simulink model "LRMate200Experimentor_Dual"  (R2015b)
settings: Solver=FixedStepDiscrete  StartTime=0.0  StopTime=inf  FixedStep=si.SolverTimeStep  RelTol=1e-3  AbsTol=1e-5
undefined symbols (not defined in the file or in its folder): si
libraries: xpcethercatlib x115, slrtlib x16, xpcnilib x10
(part 2 of 2)

== system LRMate200Experimentor_Dual/IO System/DSA System/DSA System 1/EtherCAT DSA TrqLimit ==
  In1 : Inport
  Conversion7 : DataTypeConversion
  Demux : Demux  Outputs=6
  "ToDSA J1TrqLimit " : xpcethercatlib/EtherCAT PDO Transmit   Priority=3  sig_name=Box 1 (Degital Servo Adapter).HS-OUT-AX01.AX01-HSO05  sig_offset=392  sig_type=int16  type_size=16  sig_dim=1  device_id=0  sample_time=0.000250
  ToDSA J2TrqLimit : xpcethercatlib/EtherCAT PDO Transmit   Priority=3  sig_name=Box 1 (Degital Servo Adapter).HS-OUT-AX02.AX02-HSO05  sig_offset=648  sig_type=int16  type_size=16  sig_dim=1  device_id=0  sample_time=0.000250
  ToDSA J3TrqLimit : xpcethercatlib/EtherCAT PDO Transmit   Priority=3  sig_name=Box 1 (Degital Servo Adapter).HS-OUT-AX03.AX03-HSO05  sig_offset=904  sig_type=int16  type_size=16  sig_dim=1  device_id=0  sample_time=0.000250
  ToDSA J4TrqLimit : xpcethercatlib/EtherCAT PDO Transmit   Priority=3  sig_name=Box 1 (Degital Servo Adapter).HS-OUT-AX04.AX04-HSO05  sig_offset=1160  sig_type=int16  type_size=16  sig_dim=1  device_id=0  sample_time=0.000250
  ToDSA J5TrqLimit : xpcethercatlib/EtherCAT PDO Transmit   Priority=3  sig_name=Box 2 (Degital Servo Adapter).HS-OUT-AX01.AX01-HSO05  sig_offset=2696  sig_type=int16  type_size=16  sig_dim=1  device_id=0  sample_time=0.000250
  ToDSA J6TrqLimit : xpcethercatlib/EtherCAT PDO Transmit   Priority=3  sig_name=Box 2 (Degital Servo Adapter).HS-OUT-AX02.AX02-HSO05  sig_offset=2952  sig_type=int16  type_size=16  sig_dim=1  device_id=0  sample_time=0.000250
  wires:
  In1/1 -> Conversion7/1
  Demux/1 -> "ToDSA J1TrqLimit "/1
  Demux/2 -> ToDSA J2TrqLimit/1
  Demux/3 -> ToDSA J3TrqLimit/1
  Demux/4 -> ToDSA J4TrqLimit/1
  Demux/5 -> ToDSA J5TrqLimit/1
  Demux/6 -> ToDSA J6TrqLimit/1
  Conversion7/1 -> Demux/1

== system LRMate200Experimentor_Dual/IO System/DSA System/DSA System 1/EtherCAT DSA VelOut ==
  FromDSA J1Vel : xpcethercatlib/EtherCAT PDO Receive  Priority=2  sig_name=Box 1 (Degital Servo Adapter).HS-IN-AX01.AX01-HSI10  sig_offset=472  sig_type=int32  type_size=32  sig_dim=1  device_id=0  sample_time=0.000250
  FromDSA J2Vel : xpcethercatlib/EtherCAT PDO Receive  Priority=2  sig_name=Box 1 (Degital Servo Adapter).HS-IN-AX02.AX02-HSI10  sig_offset=728  sig_type=int32  type_size=32  sig_dim=1  device_id=0  sample_time=0.000250
  FromDSA J3Vel : xpcethercatlib/EtherCAT PDO Receive  Priority=2  sig_name=Box 1 (Degital Servo Adapter).HS-IN-AX03.AX03-HSI10  sig_offset=984  sig_type=int32  type_size=32  sig_dim=1  device_id=0  sample_time=0.000250
  FromDSA J4Vel : xpcethercatlib/EtherCAT PDO Receive  Priority=2  sig_name=Box 1 (Degital Servo Adapter).HS-IN-AX04.AX04-HSI10  sig_offset=1240  sig_type=int32  type_size=32  sig_dim=1  device_id=0  sample_time=0.000250
  FromDSA J5Vel : xpcethercatlib/EtherCAT PDO Receive  Priority=2  sig_name=Box 2 (Degital Servo Adapter).HS-IN-AX01.AX01-HSI10  sig_offset=2776  sig_type=int32  type_size=32  sig_dim=1  device_id=0  sample_time=0.000250
  FromDSA J6Vel : xpcethercatlib/EtherCAT PDO Receive  Priority=2  sig_name=Box 2 (Degital Servo Adapter).HS-IN-AX02.AX02-HSI10  sig_offset=3032  sig_type=int32  type_size=32  sig_dim=1  device_id=0  sample_time=0.000250
  Mux : Mux  Inputs=6
  Rate Transition : RateTransition  OutPortSampleTime=si.tsv
  VelOut : Outport
  wires:
  FromDSA J6Vel/1 -> Mux/6
  FromDSA J4Vel/1 -> Mux/4
  FromDSA J2Vel/1 -> Mux/2
  FromDSA J5Vel/1 -> Mux/5
  FromDSA J3Vel/1 -> Mux/3
  FromDSA J1Vel/1 -> Mux/1
  Rate Transition/1 -> VelOut/1
  Mux/1 -> Rate Transition/1

== system LRMate200Experimentor_Dual/IO System/DSA System/DSA System 2/EtherCAT DSA AxEtcInfo ==
  FromDSA J1AxEtcInfo : xpcethercatlib/EtherCAT PDO Receive  Priority=2  sig_name=Box 3 (Degital Servo Adapter).NS-IN-AX01.AX01-NSI07  sig_offset=6312  sig_type=uint16  type_size=16  sig_dim=1  device_id=0  sample_time=0.000250
  FromDSA J2AxEtcInfo : xpcethercatlib/EtherCAT PDO Receive  Priority=2  sig_name=Box 3 (Degital Servo Adapter).NS-IN-AX02.AX02-NSI07  sig_offset=6504  sig_type=uint16  type_size=16  sig_dim=1  device_id=0  sample_time=0.000250
  FromDSA J3AxEtcInfo : xpcethercatlib/EtherCAT PDO Receive  Priority=2  sig_name=Box 3 (Degital Servo Adapter).NS-IN-AX03.AX03-NSI07  sig_offset=6696  sig_type=uint16  type_size=16  sig_dim=1  device_id=0  sample_time=0.000250
  FromDSA J4AxEtcInfo : xpcethercatlib/EtherCAT PDO Receive  Priority=2  sig_name=Box 3 (Degital Servo Adapter).NS-IN-AX04.AX04-NSI07  sig_offset=6888  sig_type=uint16  type_size=16  sig_dim=1  device_id=0  sample_time=0.000250
  FromDSA J5AxEtcInfo : xpcethercatlib/EtherCAT PDO Receive  Priority=2  sig_name=Box 4 (Degital Servo Adapter).NS-IN-AX01.AX01-NSI07  sig_offset=8616  sig_type=uint16  type_size=16  sig_dim=1  device_id=0  sample_time=0.000250
  FromDSA J6AxEtcInfo : xpcethercatlib/EtherCAT PDO Receive  Priority=2  sig_name=Box 4 (Degital Servo Adapter).NS-IN-AX02.AX02-NSI07  sig_offset=8808  sig_type=uint16  type_size=16  sig_dim=1  device_id=0  sample_time=0.000250
  Mux : Mux  Inputs=6
  Rate Transition : RateTransition  OutPortSampleTime=si.tsv
  AxEtcInfoOut : Outport
  wires:
  FromDSA J6AxEtcInfo/1 -> Mux/6
  FromDSA J4AxEtcInfo/1 -> Mux/4
  FromDSA J2AxEtcInfo/1 -> Mux/2
  FromDSA J5AxEtcInfo/1 -> Mux/5
  FromDSA J3AxEtcInfo/1 -> Mux/3
  FromDSA J1AxEtcInfo/1 -> Mux/1
  Mux/1 -> Rate Transition/1
  Rate Transition/1 -> AxEtcInfoOut/1

== system LRMate200Experimentor_Dual/IO System/DSA System/DSA System 2/EtherCAT DSA CurrentOut ==
  FromDSA J1Current : xpcethercatlib/EtherCAT PDO Receive  Priority=2  sig_name=Box 3 (Degital Servo Adapter).HS-IN-AX01.AX01-HSI03  sig_offset=4968  sig_type=int16  type_size=16  sig_dim=1  device_id=0  sample_time=0.000250
  FromDSA J2Current : xpcethercatlib/EtherCAT PDO Receive  Priority=2  sig_name=Box 3 (Degital Servo Adapter).HS-IN-AX02.AX02-HSI03  sig_offset=5224  sig_type=int16  type_size=16  sig_dim=1  device_id=0  sample_time=0.000250
  FromDSA J3Current : xpcethercatlib/EtherCAT PDO Receive  Priority=2  sig_name=Box 3 (Degital Servo Adapter).HS-IN-AX03.AX03-HSI03  sig_offset=5480  sig_type=int16  type_size=16  sig_dim=1  device_id=0  sample_time=0.000250
  FromDSA J4Current : xpcethercatlib/EtherCAT PDO Receive  Priority=2  sig_name=Box 3 (Degital Servo Adapter).HS-IN-AX04.AX04-HSI03  sig_offset=5736  sig_type=int16  type_size=16  sig_dim=1  device_id=0  sample_time=0.000250
  FromDSA J5Current : xpcethercatlib/EtherCAT PDO Receive  Priority=2  sig_name=Box 4 (Degital Servo Adapter).HS-IN-AX01.AX01-HSI03  sig_offset=7272  sig_type=int16  type_size=16  sig_dim=1  device_id=0  sample_time=0.000250
  FromDSA J6Current : xpcethercatlib/EtherCAT PDO Receive  Priority=2  sig_name=Box 4 (Degital Servo Adapter).HS-IN-AX02.AX02-HSI03  sig_offset=7528  sig_type=int16  type_size=16  sig_dim=1  device_id=0  sample_time=0.000250
  Mux : Mux  Inputs=6
  Rate Transition : RateTransition  OutPortSampleTime=si.tsv
  CurrentOut : Outport
  wires:
  FromDSA J6Current/1 -> Mux/6
  FromDSA J4Current/1 -> Mux/4
  FromDSA J2Current/1 -> Mux/2
  FromDSA J5Current/1 -> Mux/5
  FromDSA J3Current/1 -> Mux/3
  FromDSA J1Current/1 -> Mux/1
  Mux/1 -> Rate Transition/1
  Rate Transition/1 -> CurrentOut/1

== system LRMate200Experimentor_Dual/IO System/DSA System/DSA System 2/EtherCAT DSA IniPos ==
  FromDSA J1IniPos : xpcethercatlib/EtherCAT PDO Receive  Priority=2  sig_name=Box 3 (Degital Servo Adapter).NS-IN-AX01.AX01-NSI02  sig_offset=6232  sig_type=int32  type_size=32  sig_dim=1  device_id=0  sample_time=0.000250
  FromDSA J2IniPos : xpcethercatlib/EtherCAT PDO Receive  Priority=2  sig_name=Box 3 (Degital Servo Adapter).NS-IN-AX02.AX02-NSI02  sig_offset=6424  sig_type=int32  type_size=32  sig_dim=1  device_id=0  sample_time=0.000250
  FromDSA J3IniPos : xpcethercatlib/EtherCAT PDO Receive  Priority=2  sig_name=Box 3 (Degital Servo Adapter).NS-IN-AX03.AX03-NSI02  sig_offset=6616  sig_type=int32  type_size=32  sig_dim=1  device_id=0  sample_time=0.000250
  FromDSA J4IniPos : xpcethercatlib/EtherCAT PDO Receive  Priority=2  sig_name=Box 3 (Degital Servo Adapter).NS-IN-AX04.AX04-NSI02  sig_offset=6808  sig_type=int32  type_size=32  sig_dim=1  device_id=0  sample_time=0.000250
  FromDSA J5IniPos : xpcethercatlib/EtherCAT PDO Receive  Priority=2  sig_name=Box 4 (Degital Servo Adapter).NS-IN-AX01.AX01-NSI02  sig_offset=8536  sig_type=int32  type_size=32  sig_dim=1  device_id=0  sample_time=0.000250
  FromDSA J6IniPos : xpcethercatlib/EtherCAT PDO Receive  Priority=2  sig_name=Box 4 (Degital Servo Adapter).NS-IN-AX02.AX02-NSI02  sig_offset=8728  sig_type=int32  type_size=32  sig_dim=1  device_id=0  sample_time=0.000250
  Mux : Mux  Inputs=6
  Rate Transition : RateTransition  OutPortSampleTime=si.tsv
  ini_pos : Outport
  wires:
  FromDSA J6IniPos/1 -> Mux/6
  FromDSA J4IniPos/1 -> Mux/4
  FromDSA J2IniPos/1 -> Mux/2
  FromDSA J5IniPos/1 -> Mux/5
  FromDSA J3IniPos/1 -> Mux/3
  FromDSA J1IniPos/1 -> Mux/1
  Mux/1 -> Rate Transition/1
  Rate Transition/1 -> ini_pos/1

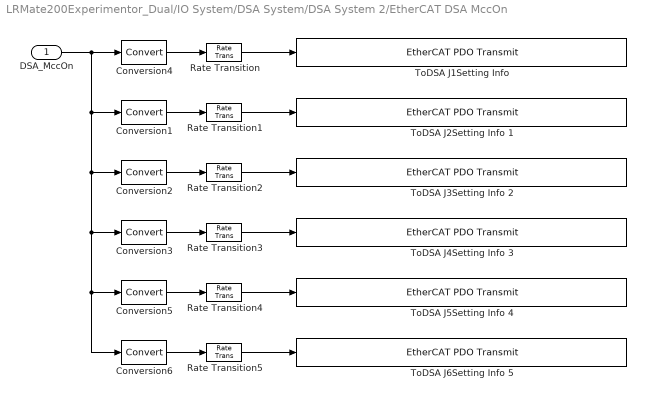
== system LRMate200Experimentor_Dual/IO System/DSA System/DSA System 2/EtherCAT DSA MccOn ==
  DSA_MccOn : Inport
  Conversion{1..6} (6 alike) : DataTypeConversion
  Rate Transition{,1..5} (6 alike) : RateTransition
  "ToDSA J1Setting Info " : xpcethercatlib/EtherCAT PDO Transmit   Priority=3  sig_name=Box 3 (Degital Servo Adapter).NS-OUT-AX01.AX01-NSO03  sig_offset=6248  sig_type=uint16  type_size=16  sig_dim=1  device_id=0  sample_time=0.000250
  ToDSA J2Setting Info 1 : xpcethercatlib/EtherCAT PDO Transmit   Priority=3  sig_name=Box 3 (Degital Servo Adapter).NS-OUT-AX02.AX02-NSO03  sig_offset=6504  sig_type=uint16  type_size=16  sig_dim=1  device_id=0  sample_time=0.000250
  ToDSA J3Setting Info 2 : xpcethercatlib/EtherCAT PDO Transmit   Priority=3  sig_name=Box 3 (Degital Servo Adapter).NS-OUT-AX03.AX03-NSO03  sig_offset=6760  sig_type=uint16  type_size=16  sig_dim=1  device_id=0  sample_time=0.000250
  ToDSA J4Setting Info 3 : xpcethercatlib/EtherCAT PDO Transmit   Priority=3  sig_name=Box 3 (Degital Servo Adapter).NS-OUT-AX04.AX04-NSO03  sig_offset=7016  sig_type=uint16  type_size=16  sig_dim=1  device_id=0  sample_time=0.000250
  ToDSA J5Setting Info 4 : xpcethercatlib/EtherCAT PDO Transmit   Priority=3  sig_name=Box 4 (Degital Servo Adapter).NS-OUT-AX01.AX01-NSO03  sig_offset=8552  sig_type=uint16  type_size=16  sig_dim=1  device_id=0  sample_time=0.000250
  ToDSA J6Setting Info 5 : xpcethercatlib/EtherCAT PDO Transmit   Priority=3  sig_name=Box 4 (Degital Servo Adapter).NS-OUT-AX02.AX02-NSO03  sig_offset=8808  sig_type=uint16  type_size=16  sig_dim=1  device_id=0  sample_time=0.000250
  wires:
  Rate Transition/1 -> "ToDSA J1Setting Info "/1
  Conversion4/1 -> Rate Transition/1
  DSA_MccOn/1 -> Conversion6/1, Conversion5/1, Conversion3/1, Conversion2/1, Conversion1/1, Conversion4/1
  Rate Transition1/1 -> ToDSA J2Setting Info 1/1
  Conversion1/1 -> Rate Transition1/1
  Rate Transition2/1 -> ToDSA J3Setting Info 2/1
  Conversion2/1 -> Rate Transition2/1
  Rate Transition3/1 -> ToDSA J4Setting Info 3/1
  Conversion3/1 -> Rate Transition3/1
  Rate Transition4/1 -> ToDSA J5Setting Info 4/1
  Conversion5/1 -> Rate Transition4/1
  Rate Transition5/1 -> ToDSA J6Setting Info 5/1
  Conversion6/1 -> Rate Transition5/1

== system LRMate200Experimentor_Dual/IO System/DSA System/DSA System 2/EtherCAT DSA PosOut ==
  FromDSA J1Pos : xpcethercatlib/EtherCAT PDO Receive  Priority=2  sig_name=Box 3 (Degital Servo Adapter).HS-IN-AX01.AX01-HSI12  sig_offset=5112  sig_type=int32  type_size=32  sig_dim=1  device_id=0  sample_time=0.000250
  FromDSA J2Pos : xpcethercatlib/EtherCAT PDO Receive  Priority=2  sig_name=Box 3 (Degital Servo Adapter).HS-IN-AX02.AX02-HSI12  sig_offset=5368  sig_type=int32  type_size=32  sig_dim=1  device_id=0  sample_time=0.000250
  FromDSA J3Pos : xpcethercatlib/EtherCAT PDO Receive  Priority=2  sig_name=Box 3 (Degital Servo Adapter).HS-IN-AX03.AX03-HSI12  sig_offset=5624  sig_type=int32  type_size=32  sig_dim=1  device_id=0  sample_time=0.000250
  FromDSA J4Pos : xpcethercatlib/EtherCAT PDO Receive  Priority=2  sig_name=Box 3 (Degital Servo Adapter).HS-IN-AX04.AX04-HSI12  sig_offset=5880  sig_type=int32  type_size=32  sig_dim=1  device_id=0  sample_time=0.000250
  FromDSA J5Pos : xpcethercatlib/EtherCAT PDO Receive  Priority=2  sig_name=Box 4 (Degital Servo Adapter).HS-IN-AX01.AX01-HSI12  sig_offset=7416  sig_type=int32  type_size=32  sig_dim=1  device_id=0  sample_time=0.000250
  FromDSA J6Pos : xpcethercatlib/EtherCAT PDO Receive  Priority=2  sig_name=Box 4 (Degital Servo Adapter).HS-IN-AX02.AX02-HSI12  sig_offset=7672  sig_type=int32  type_size=32  sig_dim=1  device_id=0  sample_time=0.000250
  Mux : Mux  Inputs=6
  Rate Transition : RateTransition  OutPortSampleTime=si.tsv
  PosOut : Outport
  wires:
  FromDSA J6Pos/1 -> Mux/6
  FromDSA J4Pos/1 -> Mux/4
  FromDSA J2Pos/1 -> Mux/2
  FromDSA J5Pos/1 -> Mux/5
  FromDSA J3Pos/1 -> Mux/3
  FromDSA J1Pos/1 -> Mux/1
  Mux/1 -> Rate Transition/1
  Rate Transition/1 -> PosOut/1

== system LRMate200Experimentor_Dual/IO System/DSA System/DSA System 2/EtherCAT DSA TrqCmd ==
  In1 : Inport
  Conversion1 : DataTypeConversion
  Demux : Demux  Outputs=6
  Rate Transition : RateTransition
  "ToDSA J1TrqCmd " : xpcethercatlib/EtherCAT PDO Transmit   Priority=3  sig_name=Box 3 (Degital Servo Adapter).HS-OUT-AX01.AX01-HSO04  sig_offset=4984  sig_type=int16  type_size=16  sig_dim=1  device_id=0  sample_time=0.000250
  ToDSA J2TrqCmd : xpcethercatlib/EtherCAT PDO Transmit   Priority=3  sig_name=Box 3 (Degital Servo Adapter).HS-OUT-AX02.AX02-HSO04  sig_offset=5240  sig_type=int16  type_size=16  sig_dim=1  device_id=0  sample_time=0.000250
  ToDSA J3TrqCmd : xpcethercatlib/EtherCAT PDO Transmit   Priority=3  sig_name=Box 3 (Degital Servo Adapter).HS-OUT-AX03.AX03-HSO04  sig_offset=5496  sig_type=int16  type_size=16  sig_dim=1  device_id=0  sample_time=0.000250
  ToDSA J4TrqCmd : xpcethercatlib/EtherCAT PDO Transmit   Priority=3  sig_name=Box 3 (Degital Servo Adapter).HS-OUT-AX04.AX04-HSO04  sig_offset=5752  sig_type=int16  type_size=16  sig_dim=1  device_id=0  sample_time=0.000250
  ToDSA J5TrqCmd : xpcethercatlib/EtherCAT PDO Transmit   Priority=3  sig_name=Box 4 (Degital Servo Adapter).HS-OUT-AX01.AX01-HSO04  sig_offset=7288  sig_type=int16  type_size=16  sig_dim=1  device_id=0  sample_time=0.000250
  ToDSA J6TrqCmd : xpcethercatlib/EtherCAT PDO Transmit   Priority=3  sig_name=Box 4 (Degital Servo Adapter).HS-OUT-AX02.AX02-HSO04  sig_offset=7544  sig_type=int16  type_size=16  sig_dim=1  device_id=0  sample_time=0.000250
  wires:
  In1/1 -> Conversion1/1
  Conversion1/1 -> Rate Transition/1
  Rate Transition/1 -> Demux/1
  Demux/1 -> "ToDSA J1TrqCmd "/1
  Demux/2 -> ToDSA J2TrqCmd/1
  Demux/3 -> ToDSA J3TrqCmd/1
  Demux/4 -> ToDSA J4TrqCmd/1
  Demux/5 -> ToDSA J5TrqCmd/1
  Demux/6 -> ToDSA J6TrqCmd/1

== system LRMate200Experimentor_Dual/IO System/DSA System/DSA System 2/EtherCAT DSA TrqCmdOut ==
  FromDSA J1TrqCmd : xpcethercatlib/EtherCAT PDO Receive  Priority=2  sig_name=Box 3 (Degital Servo Adapter).HS-IN-AX01.AX01-HSI02  sig_offset=4952  sig_type=int16  type_size=16  sig_dim=1  device_id=0  sample_time=0.000250
  FromDSA J2TrqCmd : xpcethercatlib/EtherCAT PDO Receive  Priority=2  sig_name=Box 3 (Degital Servo Adapter).HS-IN-AX02.AX02-HSI02  sig_offset=5208  sig_type=int16  type_size=16  sig_dim=1  device_id=0  sample_time=0.000250
  FromDSA J3TrqCmd2 : xpcethercatlib/EtherCAT PDO Receive  Priority=2  sig_name=Box 3 (Degital Servo Adapter).HS-IN-AX03.AX03-HSI02  sig_offset=5464  sig_type=int16  type_size=16  sig_dim=1  device_id=0  sample_time=0.000250
  FromDSA J4TrqCmd3 : xpcethercatlib/EtherCAT PDO Receive  Priority=2  sig_name=Box 3 (Degital Servo Adapter).HS-IN-AX04.AX04-HSI02  sig_offset=5720  sig_type=int16  type_size=16  sig_dim=1  device_id=0  sample_time=0.000250
  FromDSA J5TrqCmd4 : xpcethercatlib/EtherCAT PDO Receive  Priority=2  sig_name=Box 4 (Degital Servo Adapter).HS-IN-AX01.AX01-HSI02  sig_offset=7256  sig_type=int16  type_size=16  sig_dim=1  device_id=0  sample_time=0.000250
  FromDSA J6TrqCmd5 : xpcethercatlib/EtherCAT PDO Receive  Priority=2  sig_name=Box 4 (Degital Servo Adapter).HS-IN-AX02.AX02-HSI02  sig_offset=7512  sig_type=int16  type_size=16  sig_dim=1  device_id=0  sample_time=0.000250
  Mux : Mux  Inputs=6
  Rate Transition : RateTransition  OutPortSampleTime=si.tsv
  TrqCmdOut : Outport
  wires:
  FromDSA J6TrqCmd5/1 -> Mux/6
  FromDSA J4TrqCmd3/1 -> Mux/4
  FromDSA J2TrqCmd/1 -> Mux/2
  FromDSA J5TrqCmd4/1 -> Mux/5
  FromDSA J3TrqCmd2/1 -> Mux/3
  FromDSA J1TrqCmd/1 -> Mux/1
  Mux/1 -> Rate Transition/1
  Rate Transition/1 -> TrqCmdOut/1

== system LRMate200Experimentor_Dual/IO System/DSA System/DSA System 2/EtherCAT DSA TrqLimit ==
  In1 : Inport
  Conversion1 : DataTypeConversion
  Demux : Demux  Outputs=6
  "ToDSA J1TrqLimit " : xpcethercatlib/EtherCAT PDO Transmit   Priority=3  sig_name=Box 3 (Degital Servo Adapter).HS-OUT-AX01.AX01-HSO05  sig_offset=5000  sig_type=int16  type_size=16  sig_dim=1  device_id=0  sample_time=0.000250
  ToDSA J2TrqLimit : xpcethercatlib/EtherCAT PDO Transmit   Priority=3  sig_name=Box 3 (Degital Servo Adapter).HS-OUT-AX02.AX02-HSO05  sig_offset=5256  sig_type=int16  type_size=16  sig_dim=1  device_id=0  sample_time=0.000250
  ToDSA J3TrqLimit : xpcethercatlib/EtherCAT PDO Transmit   Priority=3  sig_name=Box 3 (Degital Servo Adapter).HS-OUT-AX03.AX03-HSO05  sig_offset=5512  sig_type=int16  type_size=16  sig_dim=1  device_id=0  sample_time=0.000250
  ToDSA J4TrqLimit : xpcethercatlib/EtherCAT PDO Transmit   Priority=3  sig_name=Box 3 (Degital Servo Adapter).HS-OUT-AX04.AX04-HSO05  sig_offset=5768  sig_type=int16  type_size=16  sig_dim=1  device_id=0  sample_time=0.000250
  ToDSA J5TrqLimit : xpcethercatlib/EtherCAT PDO Transmit   Priority=3  sig_name=Box 4 (Degital Servo Adapter).HS-OUT-AX01.AX01-HSO05  sig_offset=7304  sig_type=int16  type_size=16  sig_dim=1  device_id=0  sample_time=0.000250
  ToDSA J6TrqLimit : xpcethercatlib/EtherCAT PDO Transmit   Priority=3  sig_name=Box 4 (Degital Servo Adapter).HS-OUT-AX02.AX02-HSO05  sig_offset=7560  sig_type=int16  type_size=16  sig_dim=1  device_id=0  sample_time=0.000250
  wires:
  In1/1 -> Conversion1/1
  Conversion1/1 -> Demux/1
  Demux/1 -> "ToDSA J1TrqLimit "/1
  Demux/2 -> ToDSA J2TrqLimit/1
  Demux/3 -> ToDSA J3TrqLimit/1
  Demux/4 -> ToDSA J4TrqLimit/1
  Demux/5 -> ToDSA J5TrqLimit/1
  Demux/6 -> ToDSA J6TrqLimit/1

== system LRMate200Experimentor_Dual/IO System/DSA System/DSA System 2/EtherCAT DSA VelOut ==
  FromDSA J1Vel : xpcethercatlib/EtherCAT PDO Receive  Priority=2  sig_name=Box 3 (Degital Servo Adapter).HS-IN-AX01.AX01-HSI10  sig_offset=5080  sig_type=int32  type_size=32  sig_dim=1  device_id=0  sample_time=0.000250
  FromDSA J2Vel : xpcethercatlib/EtherCAT PDO Receive  Priority=2  sig_name=Box 3 (Degital Servo Adapter).HS-IN-AX02.AX02-HSI10  sig_offset=5336  sig_type=int32  type_size=32  sig_dim=1  device_id=0  sample_time=0.000250
  FromDSA J3Vel : xpcethercatlib/EtherCAT PDO Receive  Priority=2  sig_name=Box 3 (Degital Servo Adapter).HS-IN-AX03.AX03-HSI10  sig_offset=5592  sig_type=int32  type_size=32  sig_dim=1  device_id=0  sample_time=0.000250
  FromDSA J4Vel : xpcethercatlib/EtherCAT PDO Receive  Priority=2  sig_name=Box 3 (Degital Servo Adapter).HS-IN-AX04.AX04-HSI10  sig_offset=5848  sig_type=int32  type_size=32  sig_dim=1  device_id=0  sample_time=0.000250
  FromDSA J5Vel : xpcethercatlib/EtherCAT PDO Receive  Priority=2  sig_name=Box 4 (Degital Servo Adapter).HS-IN-AX01.AX01-HSI10  sig_offset=7384  sig_type=int32  type_size=32  sig_dim=1  device_id=0  sample_time=0.000250
  FromDSA J6Vel : xpcethercatlib/EtherCAT PDO Receive  Priority=2  sig_name=Box 4 (Degital Servo Adapter).HS-IN-AX02.AX02-HSI10  sig_offset=7640  sig_type=int32  type_size=32  sig_dim=1  device_id=0  sample_time=0.000250
  Mux : Mux  Inputs=6
  Rate Transition : RateTransition  OutPortSampleTime=si.tsv
  VelOut : Outport
  wires:
  FromDSA J6Vel/1 -> Mux/6
  FromDSA J4Vel/1 -> Mux/4
  FromDSA J2Vel/1 -> Mux/2
  FromDSA J5Vel/1 -> Mux/5
  FromDSA J3Vel/1 -> Mux/3
  FromDSA J1Vel/1 -> Mux/1
  Rate Transition/1 -> VelOut/1
  Mux/1 -> Rate Transition/1

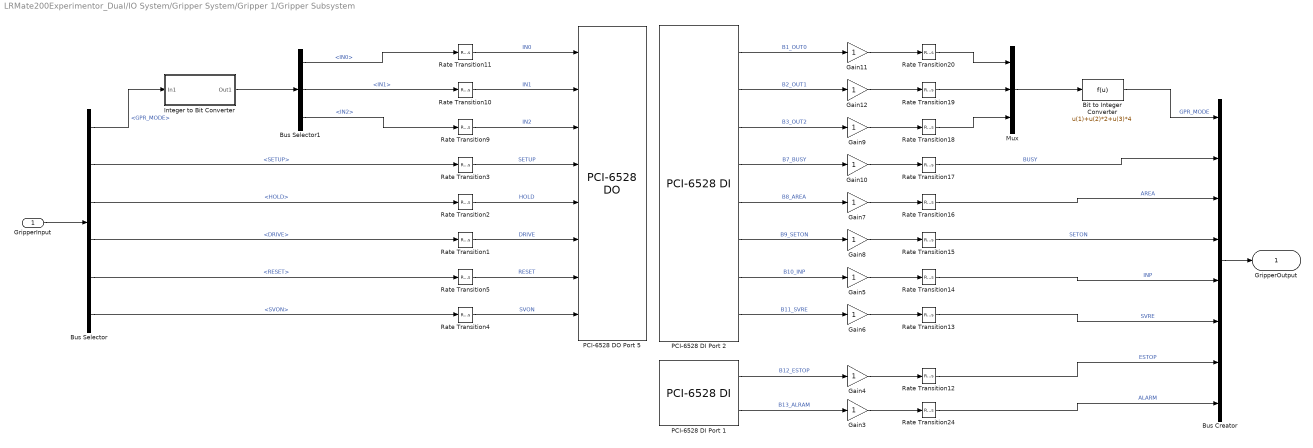
== system LRMate200Experimentor_Dual/IO System/Gripper System/Gripper 1/Gripper Subsystem ==
  GripperInput : Inport
  Bit to Integer Converter : Fcn  Expr=u(1)+u(2)*2+u(3)*4
  Bus Creator : BusCreator  Inputs=8
  Bus Selector : BusSelector  OutputSignals=GPR_MODE,SETUP,HOLD,DRIVE,RESET,SVON
  Bus Selector1 : BusSelector  OutputSignals=IN0,IN1,IN2
  Gain{3..12} (10 alike) : Gain
  Integer to Bit Converter : Subsystem  TreatAsAtomicUnit=on
  Mux : Mux  Inputs=3
  PCI-6528 DI Port 1 : xpcnilib/Digital Input/PCI-6528 DI  channel=[8 7]  port=B  filter=[0]  filtertime=0  sample=.001  slot=-1
  PCI-6528 DI Port 2 : xpcnilib/Digital Input/PCI-6528 DI  channel=[8 7 6 5 4 3 2 1]  port=C  filter=[0]  filtertime=0  sample=.001  slot=-1
  PCI-6528 DO Port 5 : xpcnilib/Digital Output/PCI-6528 DO  channel=[8 7 6 5 4 3 2 1]  port=C  reset=[1]  initValue=[0]  sample=0.001  slot=-1
  Rate Transition{1..5,9..20,24} (18 alike) : RateTransition  OutPortSampleTime=si.tsv
  GripperOutput : Outport
  wires:
  Bus Selector/4 -> Rate Transition1/1  "<DRIVE>"
  Rate Transition4/1 -> PCI-6528 DO Port 5/8  "SVON"
  Rate Transition1/1 -> PCI-6528 DO Port 5/6  "DRIVE"
  Rate Transition3/1 -> PCI-6528 DO Port 5/4  "SETUP"
  Bus Selector1/1 -> Rate Transition11/1  "<IN0>"
  Bus Selector1/2 -> Rate Transition10/1  "<IN1>"
  Bus Selector1/3 -> Rate Transition9/1  "<IN2>"
  Bus Selector/2 -> Rate Transition3/1  "<SETUP>"
  Bus Selector/3 -> Rate Transition2/1  "<HOLD>"
  Bus Selector/6 -> Rate Transition4/1  "<SVON>"
  Bus Selector/5 -> Rate Transition5/1  "<RESET>"
  Rate Transition2/1 -> PCI-6528 DO Port 5/5  "HOLD"
  Rate Transition9/1 -> PCI-6528 DO Port 5/3  "IN2"
  Rate Transition10/1 -> PCI-6528 DO Port 5/2  "IN1"
  Rate Transition11/1 -> PCI-6528 DO Port 5/1  "IN0"
  Rate Transition5/1 -> PCI-6528 DO Port 5/7  "RESET"
  GripperInput/1 -> Bus Selector/1
  Gain3/1 -> Rate Transition24/1
  PCI-6528 DI Port 2/6 -> Gain8/1  "B9_SETON"
  Bus Creator/1 -> GripperOutput/1
  Mux/1 -> Bit to Integer Converter/1
  Rate Transition18/1 -> Mux/3
  PCI-6528 DI Port 1/1 -> Gain4/1  "B12_ESTOP"
  PCI-6528 DI Port 2/3 -> Gain9/1  "B3_OUT2"
  PCI-6528 DI Port 2/4 -> Gain10/1  "B7_BUSY"
  Rate Transition20/1 -> Mux/1
  Rate Transition19/1 -> Mux/2
  PCI-6528 DI Port 2/2 -> Gain12/1  "B2_OUT1"
  Gain8/1 -> Rate Transition15/1
  Gain7/1 -> Rate Transition16/1
  PCI-6528 DI Port 2/5 -> Gain7/1  "B8_AREA"
  PCI-6528 DI Port 1/2 -> Gain3/1  "B13_ALRAM"
  Gain11/1 -> Rate Transition20/1
  Gain9/1 -> Rate Transition18/1
  Gain10/1 -> Rate Transition17/1
  Gain12/1 -> Rate Transition19/1
  Gain4/1 -> Rate Transition12/1
  Gain6/1 -> Rate Transition13/1
  PCI-6528 DI Port 2/8 -> Gain6/1  "B11_SVRE"
  PCI-6528 DI Port 2/7 -> Gain5/1  "B10_INP"
  Gain5/1 -> Rate Transition14/1
  PCI-6528 DI Port 2/1 -> Gain11/1  "B1_OUT0"
  Rate Transition16/1 -> Bus Creator/3  "AREA"
  Rate Transition17/1 -> Bus Creator/2  "BUSY"
  Rate Transition15/1 -> Bus Creator/4  "SETON"
  Bit to Integer Converter/1 -> Bus Creator/1  "GPR_MODE"
  Rate Transition13/1 -> Bus Creator/6  "SVRE"
  Rate Transition14/1 -> Bus Creator/5  "INP"
  Rate Transition12/1 -> Bus Creator/7  "ESTOP"
  Rate Transition24/1 -> Bus Creator/8  "ALARM"
  Bus Selector/1 -> Integer to Bit Converter/1(In1)  "<GPR_MODE>"
  Integer to Bit Converter/1(Out1) -> Bus Selector1/1

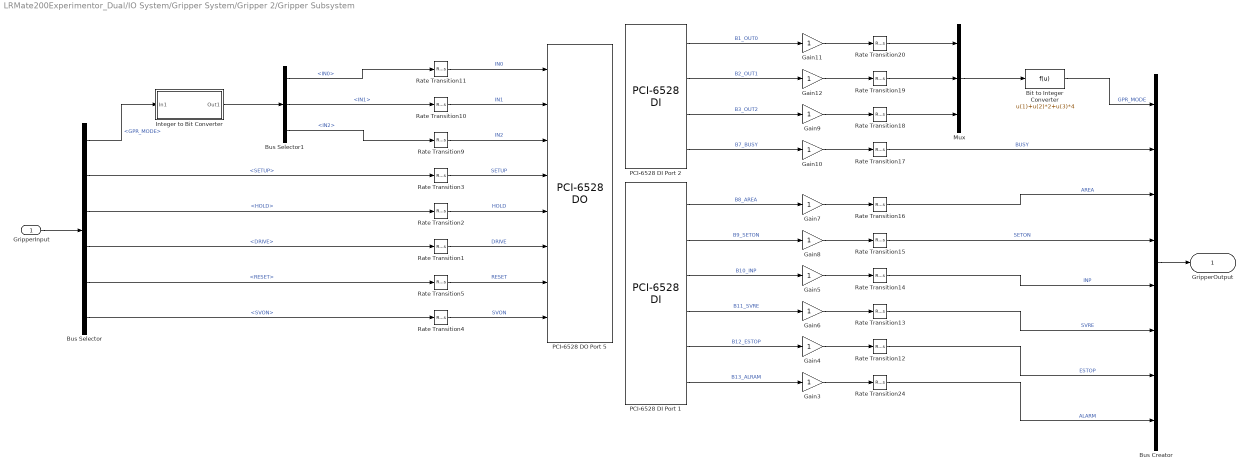
== system LRMate200Experimentor_Dual/IO System/Gripper System/Gripper 2/Gripper Subsystem ==
  GripperInput : Inport
  Bit to Integer Converter : Fcn  Expr=u(1)+u(2)*2+u(3)*4
  Bus Creator : BusCreator  Inputs=8
  Bus Selector : BusSelector  OutputSignals=GPR_MODE,SETUP,HOLD,DRIVE,RESET,SVON
  Bus Selector1 : BusSelector  OutputSignals=IN0,IN1,IN2
  Gain{3..12} (10 alike) : Gain
  Integer to Bit Converter : Subsystem  TreatAsAtomicUnit=on
  Mux : Mux  Inputs=3
  PCI-6528 DI Port 1 : xpcnilib/Digital Input/PCI-6528 DI  channel=[8 7 6 5 4 3]  port=A  filter=[0]  filtertime=0  sample=.001  slot=-1
  PCI-6528 DI Port 2 : xpcnilib/Digital Input/PCI-6528 DI  channel=[4 3 2 1]  port=B  filter=[0]  filtertime=0  sample=.001  slot=-1
  PCI-6528 DO Port 5 : xpcnilib/Digital Output/PCI-6528 DO  channel=[8 7 6 5 4 3 2 1]  port=B  reset=[1]  initValue=[0]  sample=0.001  slot=-1
  Rate Transition{1..5,9..20,24} (18 alike) : RateTransition  OutPortSampleTime=si.tsv
  GripperOutput : Outport
  wires:
  Bus Selector/4 -> Rate Transition1/1  "<DRIVE>"
  Rate Transition4/1 -> PCI-6528 DO Port 5/8  "SVON"
  Rate Transition1/1 -> PCI-6528 DO Port 5/6  "DRIVE"
  Rate Transition3/1 -> PCI-6528 DO Port 5/4  "SETUP"
  Bus Selector/2 -> Rate Transition3/1  "<SETUP>"
  Bus Selector/3 -> Rate Transition2/1  "<HOLD>"
  Bus Selector/6 -> Rate Transition4/1  "<SVON>"
  Bus Selector/5 -> Rate Transition5/1  "<RESET>"
  Rate Transition2/1 -> PCI-6528 DO Port 5/5  "HOLD"
  Rate Transition9/1 -> PCI-6528 DO Port 5/3  "IN2"
  Rate Transition10/1 -> PCI-6528 DO Port 5/2  "IN1"
  Rate Transition11/1 -> PCI-6528 DO Port 5/1  "IN0"
  Rate Transition5/1 -> PCI-6528 DO Port 5/7  "RESET"
  GripperInput/1 -> Bus Selector/1
  Gain3/1 -> Rate Transition24/1
  PCI-6528 DI Port 1/2 -> Gain8/1  "B9_SETON"
  Bus Creator/1 -> GripperOutput/1
  Mux/1 -> Bit to Integer Converter/1
  Rate Transition18/1 -> Mux/3
  PCI-6528 DI Port 1/5 -> Gain4/1  "B12_ESTOP"
  PCI-6528 DI Port 2/3 -> Gain9/1  "B3_OUT2"
  PCI-6528 DI Port 2/4 -> Gain10/1  "B7_BUSY"
  Rate Transition20/1 -> Mux/1
  Rate Transition19/1 -> Mux/2
  PCI-6528 DI Port 2/2 -> Gain12/1  "B2_OUT1"
  Gain8/1 -> Rate Transition15/1
  Gain7/1 -> Rate Transition16/1
  PCI-6528 DI Port 1/1 -> Gain7/1  "B8_AREA"
  PCI-6528 DI Port 1/6 -> Gain3/1  "B13_ALRAM"
  Gain11/1 -> Rate Transition20/1
  Gain9/1 -> Rate Transition18/1
  Gain10/1 -> Rate Transition17/1
  Gain12/1 -> Rate Transition19/1
  Gain4/1 -> Rate Transition12/1
  Gain6/1 -> Rate Transition13/1
  PCI-6528 DI Port 1/4 -> Gain6/1  "B11_SVRE"
  PCI-6528 DI Port 1/3 -> Gain5/1  "B10_INP"
  Gain5/1 -> Rate Transition14/1
  PCI-6528 DI Port 2/1 -> Gain11/1  "B1_OUT0"
  Rate Transition16/1 -> Bus Creator/3  "AREA"
  Rate Transition17/1 -> Bus Creator/2  "BUSY"
  Rate Transition15/1 -> Bus Creator/4  "SETON"
  Bit to Integer Converter/1 -> Bus Creator/1  "GPR_MODE"
  Rate Transition13/1 -> Bus Creator/6  "SVRE"
  Rate Transition14/1 -> Bus Creator/5  "INP"
  Rate Transition12/1 -> Bus Creator/7  "ESTOP"
  Rate Transition24/1 -> Bus Creator/8  "ALARM"
  Bus Selector1/1 -> Rate Transition11/1  "<IN0>"
  Bus Selector1/2 -> Rate Transition10/1  "<IN1>"
  Bus Selector1/3 -> Rate Transition9/1  "<IN2>"
  Bus Selector/1 -> Integer to Bit Converter/1(In1)  "<GPR_MODE>"
  Integer to Bit Converter/1(Out1) -> Bus Selector1/1

== system LRMate200Experimentor_Dual/IO System/Gripper System/Gripper 1/Gripper Subsystem/Integer to Bit Converter ==
  note: mod(u, 2)
  In1 : Inport
  Bus Creator : BusCreator  Inputs=3
  Fcn : Fcn  Expr=u - 2*floor(u/2)
  Fcn1 : Fcn  Expr=floor(u/2) - 2*floor(floor(u/2)/2)
  Fcn2 : Fcn  Expr=floor(u/4) - 2*floor(floor(u/4)/2)
  Out1 : Outport
  wires:
  In1/1 -> Fcn2/1, Fcn1/1, Fcn/1
  Fcn/1 -> Bus Creator/1  "IN0"
  Fcn1/1 -> Bus Creator/2  "IN1"
  Fcn2/1 -> Bus Creator/3  "IN2"
  Bus Creator/1 -> Out1/1

== system LRMate200Experimentor_Dual/IO System/Gripper System/Gripper 2/Gripper Subsystem/Integer to Bit Converter ==
  note: mod(u, 2)
  In1 : Inport
  Bus Creator : BusCreator  Inputs=3
  Fcn : Fcn  Expr=u - 2*floor(u/2)
  Fcn1 : Fcn  Expr=floor(u/2) - 2*floor(floor(u/2)/2)
  Fcn2 : Fcn  Expr=floor(u/4) - 2*floor(floor(u/4)/2)
  Out1 : Outport
  wires:
  In1/1 -> Fcn2/1, Fcn1/1, Fcn/1
  Fcn/1 -> Bus Creator/1  "IN0"
  Fcn1/1 -> Bus Creator/2  "IN1"
  Fcn2/1 -> Bus Creator/3  "IN2"
  Bus Creator/1 -> Out1/1

== matlab function LRMate200Experimentor_Dual/Dual Arm Coordination/MATLAB Function3 ==
  data: index output; TransformationM1 input; TransformationM2 input; Distance output; BASE_Z input; RADIUS input; Position output size=[6,1]; CylinGround_indexs output size=[2,1]; OFFSET input
function [index,Distance, Position,CylinGround_indexs ] = Dual_ClosestDistance_RobotandBoundary(TransformationM1, TransformationM2, BASE_Z, RADIUS, OFFSET)
%% construct cylinders for Robots
% REMINDER: add DH for robot 2, change fkine_msc for robot2 to generate
% TransforamtionM2
% for  (master robot)
p11 = TransformationM1(1:3,4,1);
p12 = TransformationM1(1:3,4,2);
p14 = TransformationM1(1:3,4,4);
p17 = TransformationM1(1:3,4,7);
C1.p1 = [0;0;BASE_Z];
C1.p2 = [0;0;0];
C1.radius = RADIUS(1);
C2.p1 = p11;
C2.p2 = p12;
C2.radius = RADIUS(2);
C3.p1 = p12;
C3.p2 = p14;
C3.radius = RADIUS(3);
C4.p1 = p14;
C4.p2 = p17;
C4.radius = RADIUS(4);
p18 = TransformationM1(1:3,4,8);
C5.p1 = (p17 - p14)*15/27 + p14; % linear function of p4 and p7
C5.p2 = p18; 
C5.radius = RADIUS(5);
% for slave robot (Stay steady) PRODUCE a offset
p21 = TransformationM2(1:3,4,1) + OFFSET;
p22 = TransformationM2(1:3,4,2) + OFFSET;
p24 = TransformationM2(1:3,4,4) + OFFSET;
p27 = TransformationM2(1:3,4,7) + OFFSET;
C6.p1 = [0;0;BASE_Z] + OFFSET;
C6.p2 = [0;0;0] + OFFSET ;
C6.radius = RADIUS(1);
C7.p1 = p21;
C7.p2 = p22;
C7.radius = RADIUS(2);
C8.p1 = p22;
C8.p2 = p24;
C8.radius = RADIUS(3);
C9.p1 = p24;
C9.p2 = p27;
C9.radius = RADIUS(4);
p28 = TransformationM2(1:3,4,8)+ OFFSET;
C10.p1 = (p27 - p24)*15/27 + p24; % linear function of p4 and p7
C10.p2 = p28; 
C10.radius = RADIUS(5);
%% check cylinders in robot. Check: 13 14 15 24 25 35; 
dmin = zeros(17,4); % change here
CylinGround_indexs = zeros(2,1); 
Position = zeros(6,1);
dmin(1,:) = [1,1,3,Distance_TwoCylinders(C1,C3)];
dmin(2,:) = [1,1,4,Distance_TwoCylinders(C1,C4)];
dmin(3,:) = [1,1,5,Distance_TwoCylinders(C1,C5)];
dmin(4,:) = [1,2,4,Distance_TwoCylinders(C2,C4)];
dmin(5,:) = [1,2,5,Distance_TwoCylinders(C2,C5)];
dmin(6,:) = [2,4,0,Distance_CylinderFloor(C4,BASE_Z)];
dmin(7,:) = [2,5,0,Distance_CylinderFloor(C5,BASE_Z)];
% addon by Yongxiang 11/17/2015
dmin(8,:) =  [1,10,5,Distance_TwoCylinders(C10,C5)];
dmin(9,:) =  [1,10,4,Distance_TwoCylinders(C10,C4)];
dmin(10,:) =  [1,10,3,Distance_TwoCylinders(C10,C3)];
dmin(11,:) =  [1,9,5,Distance_TwoCylinders(C9,C5)];
dmin(12,:) =  [1,9,4,Distance_TwoCylinders(C9,C4)];
dmin(13,:) =  [1,9,3,Distance_TwoCylinders(C9,C3)];
dmin(14,:) =  [1,8,5,Distance_TwoCylinders(C8,C5)];
dmin(15,:) =  [1,8,4,Distance_TwoCylinders(C8,C4)];
dmin(16,:) =  [1,7,5,Distance_TwoCylinders(C7,C5)];
dmin(17,:) =  [1,7,4,Distance_TwoCylinders(C7,C4)];

index1 = find(dmin(:,4) == min(dmin(:,4)));
%% find the closest cylinders and distances. 
% Distance = dmin(index,end);
% debug
% Distance = 1;
index = index1(1);
Distance = dmin(index,end);


% cylinders are:
Cylinder1 = Choose_Cylinder(C1,C2,C3,C4,C5,C6,C7,C8,C9,C10,dmin(index,2));
if dmin(index,1)==1
    Cylinder2 = Choose_Cylinder(C1,C2,C3,C4,C5,C6,C7,C8,C9,C10,dmin(index,3));
    [P1,P2] = find_clstdist_pos_consider_segment(Cylinder1,Cylinder2);
    CylinGround_indexs(1) = dmin(index,2);
    CylinGround_indexs(2) = dmin(index,3);
else % cylinder with ground has min distance
    if Cylinder1.p1(3) == min(Cylinder1.p1(3),Cylinder1.p2(3))
        P2 = Cylinder1.p1;
    else
        P2 = Cylinder1.p2;
    end
    P1 = [P2(1);P2(2);BASE_Z];
    CylinGround_indexs(1) = dmin(index,2);
    CylinGround_indexs(2) = 0;
end
Position(1:3) = P1;
Position(4:6) = P2;

end

== matlab function LRMate200Experimentor_Dual/Dual Arm Coordination/MATLAB Function4 ==
  data: F1 output; dmin input; Position input; F2 output; d0 input; dstart input; Frep output
function [F1, F2, Frep ] = RepulsiveForceGenerator(dmin, Position, d0, dstart)

P1 = Position(1:3);
P2 = Position(4:6);

% Repulsive Stiffness Gain
K = 2;  

if dmin < d0+dstart
    h = K*(d0+dstart-dmin);
else
    h = 0;
end

F1 = h/dmin *(P1 - P2);
F2 = -F1;
Frep = norm(F2);
end

== matlab function LRMate200Experimentor_Dual/Dual Arm Coordination/MATLAB Function5 ==
  data: DH_full input; TransformationM input; Position input; Index input; J output; JointPos input; DOF output
function [J,DOF ]  = Jabobian_potential_point(DH_full,TransformationM,Position,Index,JointPos)
% find Jacobian matrix for world frame, from base to witness point in
% cylinder with high freedom; J is 3*6 matrix; T is transformationM
%% Initialize
% p1 = TransformationM(1:3,4,1);
p2 = TransformationM(1:3,4,2);
p3 = TransformationM(1:3,4,3);
p5 = TransformationM(1:3,4,5);

P = Position(4:6);
index = Index(2);
n = 6;
%% Define DH parameters
% si.DH = ...   % J1           J2             J3           J4          J5            J6 
%              [  0           -1.5707963     0            0           0             0;           % Theta0 (rad)
%                 0           0              0            -0.420      0             -0.08;       % D (m)        % the last D should be -0.08 (without Gripper)
%                 0.050       0.440          0.035        0           0             0;           % A (m)
%                 -1.5707963  3.1415926      -1.5707963   1.5707963   -1.5707963    3.1415926];  % alpha (rad)           
% si.J62Gripper = 0.196;
% si.Gripper2TCP = 0.062;    
% si.ToolDH =  [  0;                                       % Theta0(rad)
%                 si.J62Gripper + si.Gripper2TCP;         % D  (m)               
%                 0;                                      % A  (m)   
%                 0];                                     % alpha (rad)
% si.Bar_DH = [0;0.1143;0.206;0];

% if index == 2 
%     dh = [0;0;norm(P-p1);0];
%     DH = [DH_full(:,1) dh zeros(4,4)];
DH = nan(4,6);
if index == 3
    
%     N = (norm(P-p2)/norm(p2-p3)<1);
%    if N==1 % here something wrong
%         dh = [0;0;norm(P-p2);0];
%         DH = [DH_full(:,1:2) dh];
%         n = 3;
%    else
%         dh = [0; -norm(P-p3); 0; 0];
%         DH = [DH_full(:,1:3) dh];
%         n = 4;
%    end
% no matter what is the N value, we consider the force is on the link 4 (n
% = 4
    dh = [0; -norm(p5-p3); 0; 0];
    DH = [DH_full(:,1:3) dh];
    n = 4;


elseif index == 4
    dh = [0; -norm(P-p5); 0; 3.1415926];
    DH = [DH_full(:,1:5) dh];
    n = 6;
elseif index == 5
    dh = [0; -0.1905; sqrt(norm(P-p5).^2 -0.1905^2); 3.1415926];
    DH = [DH_full(:,1:5) dh];
    n = 6;
else

    n = 6;
    DH = DH_full(:,1:6);
end

%% Transformation M
T = nan(4,4,n);
Tr = eye(4,4);
for i=1:n
    q = JointPos(i) + DH(1,i);
    Tr = Tr * [cos(q)      -sin(q)*cos(DH(4,i))    sin(q)*sin(DH(4,i))      DH(3,i)*cos(q);
               sin(q)      cos(q)*cos(DH(4,i))     -cos(q)*sin(DH(4,i))     sin(q)*DH(3,i);
               0           sin(DH(4,i))            cos(DH(4,i))             DH(2,i);
               0           0                       0                        1];
    T(:,:,i) = Tr;
end

%% Jacobian Matrix
J = zeros(6,6);
J(:,1) = [cross( [0;0;0] - T(1:3,4,n), [0;0;1] ); [0;0;1]];
for i=1:n-1
    J(:,i+1)=[cross( T(1:3,4,i) - T(1:3,4,n), T(1:3,3,i) ); T(1:3,3,i)];
end
% if n ==6
%     J = JacobianM;
% end
DOF = n;
% RANK = rank(J(:,1:n));
end
